simulink model "simkalman2"  (R2017b)
settings: Solver=ode4  StartTime=0.0  StopTime=10.0  FixedStep=Ts  MaxStep=0.01  RelTol=1e-3  EnableMultiTasking=on
values from neighbouring files (symbols this model uses):
  A = [1 0 0 0 0.01 1 0 0 -9.79521061044e-05 -0.0195804527741 1.00293856318 0.587413583222 ... (16 elements, 4x4)]    [diskretnySM2.mat]    (also in simdiskkyvadlo.m = expm(Ac*Ts); sysd.mat = [1 0 0 0 0.01 1 0 0 -9.7856100623e-05 -0.0195420736082 0.997; sysd2.mat)
  b = 0.1    [funkciadynamiky.m]    (also in param.mat; simnelinkyvadlo.m; simnelinkyvadlo_mine.m)
  B = [0.00012496859202 0.0249916014216 -0.000624057760604 -0.124748042648]    [diskretnySM2.mat]    (also in simdiskkyvadlo.m = Ac\(A-eye(length(A)))*Bc; sysd.mat = [0.000124948203496 0.0249834509022 0.000623446104887 0.12450; sysd2.mat)
  C = [1  0  0  0; 0  0  1  0]    [diskretnySM2.mat]    (also in sysd.mat; sysd2.mat)
  D = [0 0]    [diskretnySM2.mat]    (also in sysd.mat; sysd2.mat)
  dx0 = x0-xlin    [kalmankyvadlo.m]    (also in simEKFkyvadlo.m; simKFkyvadlo.m = zeros(nx,1); simdiskkyvadlo.m = [0;0;0;0]; simlinkyvadlo.m = [0;0;-pi/6;0])
  g = 9.81    [funkciadynamiky.m]    (also in param.mat; simnelinkyvadlo.m; simnelinkyvadlo_mine.m)
  l = 0.2    [funkciadynamiky.m]    (also in param.mat; simnelinkyvadlo.m; simnelinkyvadlo_mine.m)
  m1 = 0.4    [funkciadynamiky.m]    (also in param.mat; simnelinkyvadlo.m; simnelinkyvadlo_mine.m)
  m2 = 0.08    [funkciadynamiky.m]    (also in param.mat; simnelinkyvadlo.m; simnelinkyvadlo_mine.m)
  Q = diag(w_var)    [simEKFkyvadlo.m]    (also in simKFkyvadlo.m)
  R = diag(v_var)    [simEKFkyvadlo.m]    (also in simKFkyvadlo.m)
  Ts = 0.01    [funkciadynamiky.m]    (also in kalmankyvadlo.m; simdiskkyvadlo.m; simnelinkyvadlo_mine.m; sysd.mat)
  ulin = 0    [kalmankyvadlo.m]    (also in linearizacia.m)
  x0 = [0;0;5*pi/6;0]    [kalmankyvadlo.m]    (also in simEKFkyvadlo.m = [0;0;0;0]; simKFkyvadlo.m = [0;0;7*pi/8;0]; simnelinkyvadlo.m = [0;0;pi/6;0]; simnelinkyvadlo_mine.m = [0;0;pi/6;0])
  xlin = [0;0;pi;0]    [kalmankyvadlo.m]    (also in linearizacia.m = [0 0 pi 0]; simEKFkyvadlo.m; simKFkyvadlo.m)
  ylin = C*xlin    [kalmankyvadlo.m]
undefined symbols (not defined in the file or in its folder): Discrete, Time
libraries: simulink x3, ctrlSharedLib x1
settings Model: Creator=UAMAI-LENOVO  LastModifiedBy=gulan
settings DataIOCC: LimitDataPoints=on  SaveFormat=Array
settings OptimizationCC: LifeSpan=inf
settings DebuggingCC: SFUnexpectedBacktrackingDiag=warning  SFNoUnconditionalDefaultTransitionDiag=warning  SFExecutionAtInitializationDiag=none
settings HardwareCC: ProdBitPerPointer=32  ProdBitPerSizeT=32  ProdBitPerPtrDiffT=32  ProdLargestAtomicFloat=None  ProdIntDivRoundTo=Undefined  ProdEndianess=Unspecified  ProdWordSize=32  ProdHWDeviceType=32-bit Generic
settings ModelReferenceCC: PropagateSignalLabelsOutOfModel=off
settings CodeAppCC: StateflowObjectComments=on
settings GRTTargetCC: TargetLangStandard=C89/C90 (ANSI)  GeneratePreprocessorConditionals=Disable all
settings ConfigComp: CovMetricSettings=dw  CovHtmlReporting=on  CovSaveCumulativeToWorkspaceVar=on  CovSaveSingleToWorkspaceVar=on  CovExternalEMLEnable=off

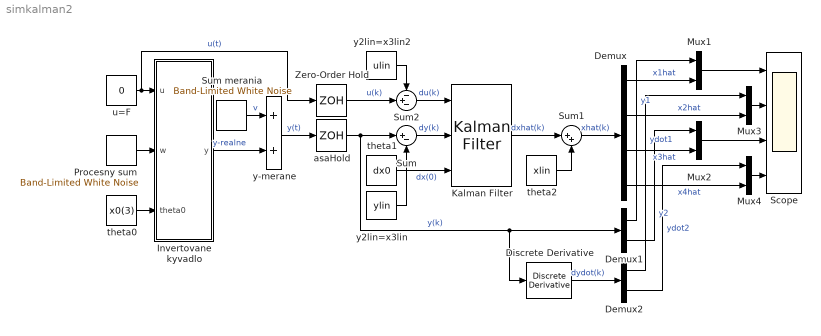
== system simkalman2 ==
  " Scope" : Scope  NumInputPorts=4
  " y-merane " : Sum
  Demux : Demux
  Demux1 : Demux  Outputs=2
  Demux2 : Demux  Outputs=2
  Discrete Derivative : simulink/Discrete/Discrete Derivative  gainval=1.0  ICPrevScaledInput=x0([1 3])/Ts  OutMin=[]  OutMax=[]  OutDataType=fixdt(1, 16)  OutScaling=2^-10  DoSatur=off
  Invertovane kyvadlo : Subsystem
  Kalman Filter : ctrlSharedLib/Kalman Filter  TimeDomain=Discrete-Time  UseCurrentEstimator=on  ModelSource=Individual A, B, C, D matrices  ModelSourceVariable=sysd  A=A  B=B  C=C  D=D  NumberOfStates=1  NumberOfInputs=1  NumberOfOutputs=1  InitialEstimateSource=Input port  X0=dx0  P0=10  UseK=off  UseGH=off  NumberOfProcessNoiseInputs=1  G=1  TimeInvariantG=on  H=0  TimeInvariantH=on  Q=diag([0 0 0 Q])  TimeInvariantQ=on  R=R  TimeInvariantR=on  N=0  TimeInvariantN=on  AddInputPort=on  AddEnablePort=off  OutputEstimatedY=off  OutputP=off  Ts=-1
      settings: SourceProductBaseCode=CT
  Mux{1..4} (4 alike) : Mux  Inputs=2
  Procesny sum : simulink/Sources/Band-Limited White Noise  Cov=Q*Ts  Ts=Ts  seed=[23341]
  Sum : Sum  Inputs=|+-
  Sum merania : simulink/Sources/Band-Limited White Noise  Cov=R*Ts  Ts=Ts  seed=[12347]
  Sum1 : Sum  Inputs=|++
  Sum2 : Sum  Inputs=-+-
  Zero-Order Hold : ZeroOrderHold  SampleTime=Ts
  asaHold : ZeroOrderHold  SampleTime=Ts
  theta0 : Constant  Value=x0(3)
  theta1 : Constant  Value=dx0
  theta2 : Constant  Value=xlin
  u=F : Constant  Value=0
  y2lin=x3lin : Constant  Value=ylin
  y2lin=x3lin2 : Constant  Value=ulin
  wires:
  theta0/1 -> Invertovane kyvadlo/3(theta0)
  u=F/1 -> Zero-Order Hold/1, Invertovane kyvadlo/1(u)  "u(t)"
  Sum merania/1 -> " y-merane "/1  "v"
  Invertovane kyvadlo/1(y) -> " y-merane "/2  "y-realne"
  Kalman Filter/1 -> Sum1/1  "dxhat(k)"
  asaHold/1 -> Discrete Derivative/1, Demux1/1, Sum/1  "y(k)"
  Zero-Order Hold/1 -> Sum2/2  "u(k)"
  y2lin=x3lin/1 -> Sum/2
  Procesny sum/1 -> Invertovane kyvadlo/2(w)
  theta1/1 -> Kalman Filter/3  "dx(0)"
  Mux1/1 -> " Scope"/1
  Mux2/1 -> " Scope"/3
  theta2/1 -> Sum1/2
  Sum1/1 -> Demux/1  "xhat(k)"
  Discrete Derivative/1 -> Demux2/1  "dydot(k)"
  Demux/1 -> Mux1/2  "x1hat"
  Mux3/1 -> " Scope"/2
  Demux2/1 -> Mux3/1  "ydot1"
  Demux/2 -> Mux3/2  "x2hat"
  Demux/3 -> Mux2/2  "x3hat"
  Demux1/2 -> Mux2/1  "y2"
  Mux4/1 -> " Scope"/4
  Demux/4 -> Mux4/2  "x4hat"
  Demux2/2 -> Mux4/1  "ydot2"
  " y-merane "/1 -> asaHold/1  "y(t)"
  Sum/1 -> Kalman Filter/2  "dy(k)"
  Sum2/1 -> Kalman Filter/1  "du(k)"
  y2lin=x3lin2/1 -> Sum2/1
  Demux1/1 -> Mux1/1  "y1"

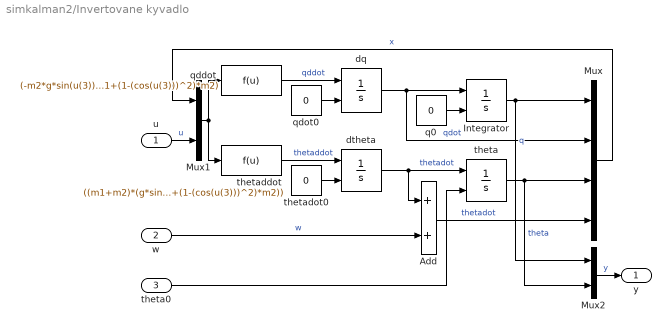
== system simkalman2/Invertovane kyvadlo ==
  u : Inport
  w : Inport  Port=2
  theta0 : Inport  Port=3
  Add : Sum
  Integrator : Integrator  InitialConditionSource=external
  Mux : Mux
  Mux1 : Mux  Inputs=2
  Mux2 : Mux  Inputs=2
  dq : Integrator  InitialConditionSource=external
  dtheta : Integrator  InitialConditionSource=external
  q0 : Constant  Value=0
  qddot : Fcn  Expr=(-m2*g*sin(u(3))*cos(u(3))+m2*l*((u(4))^2)*sin(u(3))+b*m2*u(4)*cos(u(3))+u(5))/(m1+(1-(cos(u(3)))^2)*m2)
  qdot0 : Constant  Value=0
  theta : Integrator  InitialConditionSource=external
  thetaddot : Fcn  Expr=((m1+m2)*(g*sin(u(3))-b*u(4))-(m2*l*((u(4))^2)*sin(u(3))+u(5))*cos(u(3)))/(l*(m1+(1-(cos(u(3)))^2)*m2))
  thetadot0 : Constant  Value=0
  y : Outport
  wires:
  dq/1 -> Mux/2, Integrator/1  "qdot"
  dtheta/1 -> Add/1, theta/1  "thetadot"
  Integrator/1 -> Mux/1, Mux2/1  "q"
  theta/1 -> Mux/3, Mux2/2  "theta"
  qddot/1 -> dq/1  "qddot"
  thetaddot/1 -> dtheta/1  "thetaddot"
  qdot0/1 -> dq/2
  q0/1 -> Integrator/2
  thetadot0/1 -> dtheta/2
  Mux/1 -> Mux1/1  "x"
  Mux1/1 -> thetaddot/1, qddot/1
  theta0/1 -> theta/2
  Mux2/1 -> y/1  "y"
  u/1 -> Mux1/2  "u"
  Add/1 -> Mux/4  "thetadot"
  w/1 -> Add/2  "w"
